simulink model "dsppluck"  (Simulink 6.0)
settings: Solver=FixedStepDiscrete  StartTime=0.0  StopTime=40/16  RelTol=1e-3
undefined symbols (not defined in the file or in its folder): sound, y_pluck
libraries: dspbuff3 x2, simulink x2, dspindex x2, dspsigops x1, dspsigattribs x1, dspsnks4 x1
settings Model: Creator=orofinod  LastModifiedBy=schim  ProdHWDeviceType=Specified
settings DataIOCC: SaveOutput=off  SaveTime=off  SignalLoggingName=sigsOut
settings OptimizationCC: InlineInvariantSignals=off
settings DebuggingCC: CheckExecutionContextPreStartOutputMsg=on  CheckExecutionContextRuntimeOutputMsg=on  SolverPrmCheckMsg=none
settings HardwareCC: ProdBitPerShort=32  ProdBitPerInt=16  ProdHWDeviceType=Specified
settings RTWCC: GenCodeOnly=on
settings SFSimCC: SFSimApplyToAllLibs=on  SFSimBuildMode=Incremental

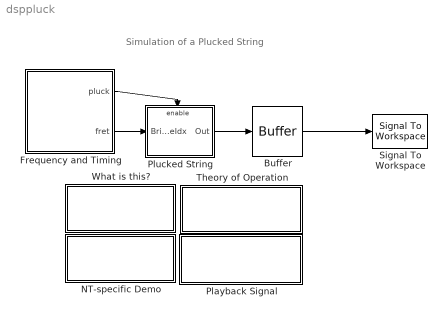
== system dsppluck ==
  note: Simulation of a Plucked String
  Buffer : dspbuff3/Buffer  N=128  V=0  ic=0
  Frequency and Timing : Subsystem  PropExecContextAcrossSSBoundary=on  mask{ptime=[0 5000 7500 10000 15000], fret=[30 14 14 23 8], Ts=1/16000}
      mask prompts: ptime "Pluck time indices:"; fret "Fret position:"; Ts "Sample time:"
      mask init:
      | % Fret position (frequency) signal
      | p=ptime(:); q=ones(size(p)).*fret(:);
      | p=p(:); q=q(:);
      | freq.time=p*Ts;
      | freq.signals.values=uint16(q);
      | freq.signals.dimensions=1;
      | 
      | % Pluck timing (enable) signal
      | p=ptime(:); p=p(2:end); q=ones(size(p));
      | p=[p p+1]'; p=[1;p(:)];
      | q=[zeros(size(q)) q]'; q=[1;q(:)];
      | ena.time=p*Ts;
      | ena.signals.values=boolean(q);
      | ena.signals.dimensions=1;
      mask Display: disp('Instrument');
  NT-specific Demo : Subsystem  PropExecContextAcrossSSBoundary=on
      settings: OpenFcn=dsppluck_win32
      mask Type: NT-only Demo
      mask Display: disp('PC/Windows\nDemo')
  Playback Signal : Subsystem  StopFcn=sound(double(y_pluck),16000);  PropExecContextAcrossSSBoundary=on
      settings: OpenFcn=|
      | if exist('y_pluck','var'),
      |    sound(double(y_pluck),16000);
      | else
      |    errordlg('Run model before playing.', ...
      |                'Signal Processing Blockset Demo Error');
      | end
      mask Type: Original Signal
      mask Display: disp('Playback\nSignal')
  Plucked String : Subsystem  TreatAsAtomicUnit=on  PropExecContextAcrossSSBoundary=on  mask(Plucked String Simulator){SLen=35, H=single(-[.25 .5 .25]), PPt=30, PickupIdx=30}
      mask prompts: SLen "String length, L (number of samples):"; H "Reflection filter (FIR):"; PPt "Pluck point, P (0 < P <= L):"; PickupIdx "Pickup index, i (0 < i <= L):"
      mask help:
      | Simulates a plucked string.  Input signal is a scalar integer value indicating the placement of the "bridge", e.g., it sets the frequency of the output.  Lower numbers lead to higher frequencies, and this must be <= L, the length of the delay line.
      |
      | String Length is a relative measure, specified in number of discrete samples, which is related to the length of the digital delay line.  It must be > 3 based on the reflection filter being used.
      |
      | Pluck Point is the position, in samples, along the string at which the displacement is centered.  This must be less than or equal to the string length.
      |
      | Pickup Index is the position,  in samples, at which the "vibration" is "sampled" to determine the output signal.
      mask init:
      | % [LtInit,RtInit] = dspblkpluck(SLen,PPt,H);
      | %
      | % pluck position is given as a sample count
      | % create triangular waveform for initialization
      | x = [ (0:floor(PPt))./PPt, ...
      |       (SLen-1-((floor(PPt)+1):(SLen-1)))./(SLen-1-PPt) ];
      | 
      | % Because initial velocity profile is flat,
      | % initial displacement profile is equal in
      | % leftgoing and rightgoing waves.
      | %
      | % Make right-going delay-line long enough to
      | % hold refl filter points centered at the end
      | % point (for calculating zero-phase reflection)
      | LtInit  = x/2;
      | RtInit = [x/2, zeros(1, length(H) - floor(length(H)/2))];
      mask Help: web(dspbhelp);
      mask Display: disp('Digital\nWaveguide\nSynthesis')
  Signal To Workspace : dspsnks4/Signal To Workspace  VariableName=y_pluck  FrameMode=Concatenate frames (2-D array)
      settings: FixptAsFi=off
  Theory of Operation : Subsystem  PropExecContextAcrossSSBoundary=on
      settings: OpenFcn=helpview(fullfile(matlabroot,'toolbox','dspblks','dspdemos','dsppluck.html'))
      mask Type: Theory of Operation
      mask Display: disp('Theory of\nOperation')
  What is this? : Subsystem  PropExecContextAcrossSSBoundary=on
      mask Type: Frame-Based Simulation Info
      mask Display: disp('What is this?')
  wires:
  Plucked String/1(Out) -> Buffer/1
  Frequency and Timing/2(fret) -> Plucked String/1(BridgeIdx)
  Buffer/1 -> Signal To Workspace/1
  Frequency and Timing/1(pluck) -> Plucked String/Enable

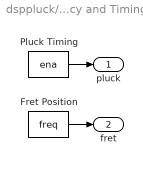
== system dsppluck/Frequency and Timing ==
  Fret Position : FromWorkspace  VariableName=freq  SampleTime=Ts  Interpolate=off  OutputAfterFinalValue=Holding final value
  Pluck Timing : FromWorkspace  VariableName=ena  SampleTime=Ts  Interpolate=off  OutputAfterFinalValue=Holding final value
  pluck : Outport
  fret : Outport  Port=2
  wires:
  Pluck Timing/1 -> pluck/1
  Fret Position/1 -> fret/1

== system dsppluck/NT-specific Demo ==

== system dsppluck/Playback Signal ==

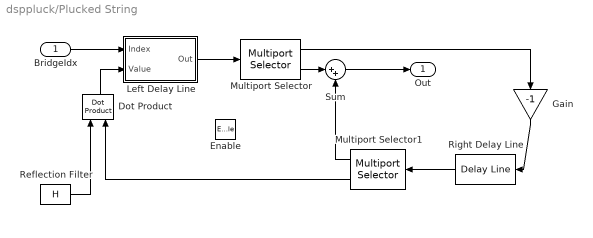
== system dsppluck/Plucked String ==
  BridgeIdx : Inport  LatchInput=off
  Enable : EnablePort  StatesWhenEnabling=reset  ZeroCross=off
  Dot Product : simulink/Math Operations/Dot Product  Orientation=up  OutDataType=sfix(16)  OutScaling=2^-10  DoSatur=off
  Gain : Gain  Orientation=down  Gain=-1  SaturateOnIntegerOverflow=on
  Left Delay Line : Subsystem  PropExecContextAcrossSSBoundary=on  mask(Variable Delay Line){siz=length(LtInit), ic=LtInit}
      mask prompts: siz "Delay line size:"; ic "Initial conditions:"
      mask help:
      | Shift out delay line contents and store input data into delay line at point specified by the Index port.
      |
      | Index port expects a 1-based index.
      mask Help: web(dspbhelp);
      mask Display: disp('Variable\nDelay\nLine');
  Multiport Selector : dspindex/Multiport Selector  rowsOrCols=Rows  idxCellArray={1, PickupIdx}  idxErrMode=Clip Index
  Multiport Selector1 : dspindex/Multiport Selector  Orientation=left  rowsOrCols=Rows  idxCellArray={PickupIdx, 1:length(H)}  idxErrMode=Clip Index
  Reflection Filter : Constant  Value=H  VectorParams1D=off
  Right Delay Line : dspbuff3/Delay Line  Orientation=left  siz=length(RtInit)  ic=RtInit  directfeed=off
  Sum : Sum  Inputs=|++  SaturateOnIntegerOverflow=on  InputSameDT=on
  Out : Outport
  wires:
  Sum/1 -> Out/1
  BridgeIdx/1 -> Left Delay Line/1(Index)
  Dot Product/1 -> Left Delay Line/2(Value)
  Gain/1 -> Right Delay Line/1
  Multiport Selector/1 -> Gain/1
  Right Delay Line/1 -> Multiport Selector1/1
  Left Delay Line/1(Out) -> Multiport Selector/1
  Reflection Filter/1 -> Dot Product/1
  Multiport Selector/2 -> Sum/1
  Multiport Selector1/2 -> Dot Product/2
  Multiport Selector1/1 -> Sum/2

== system dsppluck/Theory of Operation ==
  note: This is a simulation of a plucked string that employs digital
      | waveguide synthesis.  An on-line textbook, entitled:
      |        Digital Waveguide Modeling of Musical Instruments
      | authored by Julius O. Smith III is available, last we checked, at:
      |        http://www-ccrma.stanford.edu/~jos/waveguide/
      | and covers significant background related to digital waveguides.
      |
      | The Harmony Central website also provides very useful
      | background information on a variety of related topics:
      |     http://www.harmony-central.com/Synth/Articles/Physical_Modeling/
      |
      | This Simulink implementation is based largely on an original
      | M-file implementation available from Daniel Ellis, at:
      |       http://www.ee.columbia.edu/~dpwe/resources/matlab

== system dsppluck/What is this? ==
  note: This simulation demonstrates the use of digital
      | waveguide synthesis for a plucked string.
      |
      | Run the simulation until it completes (approx.
      | 2.5 seconds of simulation time), then the result
      | will be automatically played back using the sound
      | command.  If you wish to replay the output, just
      | double-click the "Playback Signal" block.
      |
      | To see the implementation, be sure to "Look Under"
      | the "Digital Waveguide Synthesis" block by selecting
      | the block and either hitting "ctrl+u", or right clicking
      | on the block and selecting "Look Under Mask."

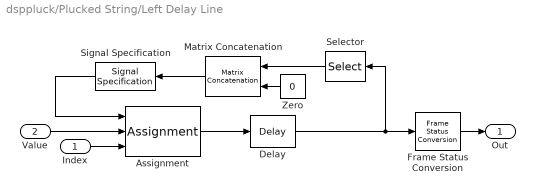
== system dsppluck/Plucked String/Left Delay Line ==
  Index : Inport  LatchInput=off
  Value : Inport  Port=2  LatchInput=off
  Assignment : Assignment  ElementSrc=External  Columns=-1
  Delay : dspsigops/Delay  dly_unit=Samples  delay=1  ic_detail=on  dif_ic_for_ch=on  dif_ic_for_dly=off  ic=ic  reset_popup=None
  Frame Status Conversion : dspsigattribs/Frame Status Conversion  growRefPort=off  outframe=Frame-based
  Matrix Concatenation : simulink/Math Operations/Matrix Concatenation  Orientation=left  numInports=2  catMethod=Vertical
  Selector : Selector  Orientation=left  Elements=2:siz  InputPortWidth=siz
  Signal Specification : SignalSpecification  Orientation=left  Dimensions=siz
  Zero : Constant  Orientation=left  Value=0  VectorParams1D=off
  Out : Outport
  wires:
  Assignment/1 -> Delay/1
  Zero/1 -> Matrix Concatenation/2
  Matrix Concatenation/1 -> Signal Specification/1
  Signal Specification/1 -> Assignment/1
  Selector/1 -> Matrix Concatenation/1
  Value/1 -> Assignment/2
  Index/1 -> Assignment/3
  Delay/1 -> Selector/1, Frame Status Conversion/1
  Frame Status Conversion/1 -> Out/1
